simulink model "RWcontrol"  (R2022a)
settings: Solver=VariableStepAuto  StartTime=0.0  StopTime=10.0  RelTol=1e-3
undefined symbols (not defined in the file): a, b, c, D, J, Kt, Ra, Tc
settings Model: Creator=sokse  LastModifiedBy=sokse

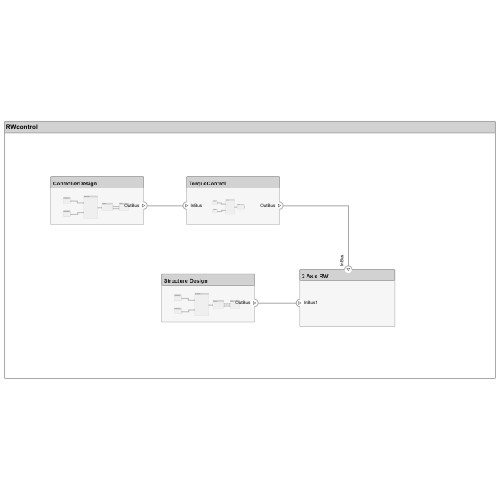
[thumbnail: Simulink's stored preview of the top-level diagram]
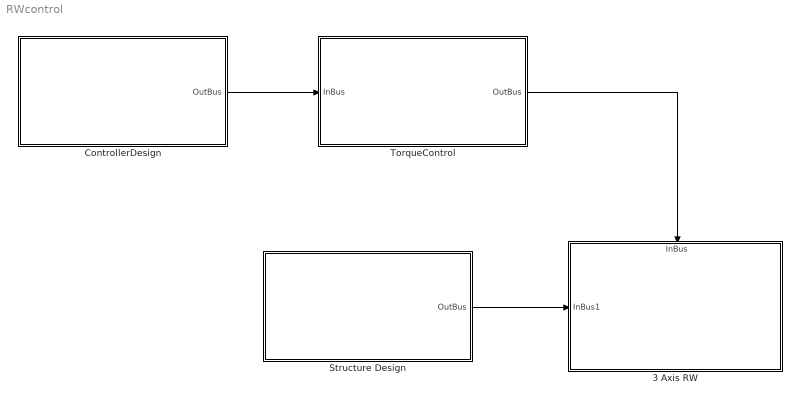
== system RWcontrol ==
  "3 Axis RW " : Subsystem
      settings: PortSchema="{\"entries\":[{\"content\":{\"headerSize\":26,\"margin\":15,\"minimumSpacing\":25,\"sides\":[{\"content\":{\"connectorIds\":[\"In1\"]},\"type\":\"ConnectorPlacement.EquallySpacedRectSide\",\"uuid\":\"5a3ed42f-ef60-4d5f-9f38-8a8f512792d6\"},{\"content\":{\"connectorIds\":[],\"side\":\"RIGHT\"},\"type\":\"ConnectorPlacement.EquallySpacedRectSide\",\"uuid\":\"59ceac5d-16f1-41c0-9a71-456f9fb7ce18\"},{\"content\":{\"connectorIds\":[\"In2\"],\"side\":\"TOP\"},\"type\":\"ConnectorPlacement.EquallySpacedRectSide\",\"uuid\":\"4a3f00af-2f72-40aa-9bae-562563b835ca\"}]},\"type\":\"ConnectorPlacement.EquallySpacedConnector\",\"uuid\":\"b5549df5-2814-423d-9e67-fe282ba68aba\"}],\"packageUris\":[\"http://schema.mathworks.com/mf0/Connector/R2020b\"],\"version\":\"1.0\"}"
  ControllerDesign : Subsystem
      settings: PortSchema="{\"entries\":[{\"content\":{\"headerSize\":26,\"margin\":15,\"minimumSpacing\":25,\"sides\":[{\"content\":{\"connectorIds\":[]},\"type\":\"ConnectorPlacement.EquallySpacedRectSide\",\"uuid\":\"5a3ed42f-ef60-4d5f-9f38-8a8f512792d6\"},{\"content\":{\"connectorIds\":[\"Out1\"],\"side\":\"RIGHT\"},\"type\":\"ConnectorPlacement.EquallySpacedRectSide\",\"uuid\":\"59ceac5d-16f1-41c0-9a71-456f9fb7ce18\"},{\"content\":{\"connectorIds\":[],\"side\":\"TOP\"},\"type\":\"ConnectorPlacement.EquallySpacedRectSide\",\"uuid\":\"4a3f00af-2f72-40aa-9bae-562563b835ca\"}]},\"type\":\"ConnectorPlacement.EquallySpacedConnector\",\"uuid\":\"b5549df5-2814-423d-9e67-fe282ba68aba\"}],\"packageUris\":[\"http://schema.mathworks.com/mf0/Connector/R2020b\"],\"version\":\"1.0\"}"
  Structure Design : Subsystem
      settings: PortSchema="{\"entries\":[{\"content\":{\"headerSize\":26,\"margin\":15,\"minimumSpacing\":25,\"sides\":[{\"content\":{\"connectorIds\":[]},\"type\":\"ConnectorPlacement.EquallySpacedRectSide\",\"uuid\":\"5a3ed42f-ef60-4d5f-9f38-8a8f512792d6\"},{\"content\":{\"connectorIds\":[\"Out1\"],\"side\":\"RIGHT\"},\"type\":\"ConnectorPlacement.EquallySpacedRectSide\",\"uuid\":\"59ceac5d-16f1-41c0-9a71-456f9fb7ce18\"},{\"content\":{\"connectorIds\":[],\"side\":\"TOP\"},\"type\":\"ConnectorPlacement.EquallySpacedRectSide\",\"uuid\":\"4a3f00af-2f72-40aa-9bae-562563b835ca\"}]},\"type\":\"ConnectorPlacement.EquallySpacedConnector\",\"uuid\":\"b5549df5-2814-423d-9e67-fe282ba68aba\"}],\"packageUris\":[\"http://schema.mathworks.com/mf0/Connector/R2020b\"],\"version\":\"1.0\"}"
  TorqueControl : Subsystem
      settings: PortSchema="{\"entries\":[{\"content\":{\"headerSize\":26,\"margin\":15,\"minimumSpacing\":25,\"sides\":[{\"content\":{\"connectorIds\":[\"In1\"]},\"type\":\"ConnectorPlacement.EquallySpacedRectSide\",\"uuid\":\"5a3ed42f-ef60-4d5f-9f38-8a8f512792d6\"},{\"content\":{\"connectorIds\":[\"Out1\"],\"side\":\"RIGHT\"},\"type\":\"ConnectorPlacement.EquallySpacedRectSide\",\"uuid\":\"59ceac5d-16f1-41c0-9a71-456f9fb7ce18\"},{\"content\":{\"connectorIds\":[],\"side\":\"TOP\"},\"type\":\"ConnectorPlacement.EquallySpacedRectSide\",\"uuid\":\"4a3f00af-2f72-40aa-9bae-562563b835ca\"}]},\"type\":\"ConnectorPlacement.EquallySpacedConnector\",\"uuid\":\"b5549df5-2814-423d-9e67-fe282ba68aba\"}],\"packageUris\":[\"http://schema.mathworks.com/mf0/Connector/R2020b\"],\"version\":\"1.0\"}"
  wires:
  ControllerDesign/1(OutBus) -> TorqueControl/1(InBus)
  TorqueControl/1(OutBus) -> "3 Axis RW "/2(InBus)
  Structure Design/1(OutBus) -> "3 Axis RW "/1(InBus1)

== system RWcontrol/3 Axis RW  ==
  Bus Element In2 : Inport  PortName=InBus1
  Bus Element In1 : Inport  Port=2  PortName=InBus

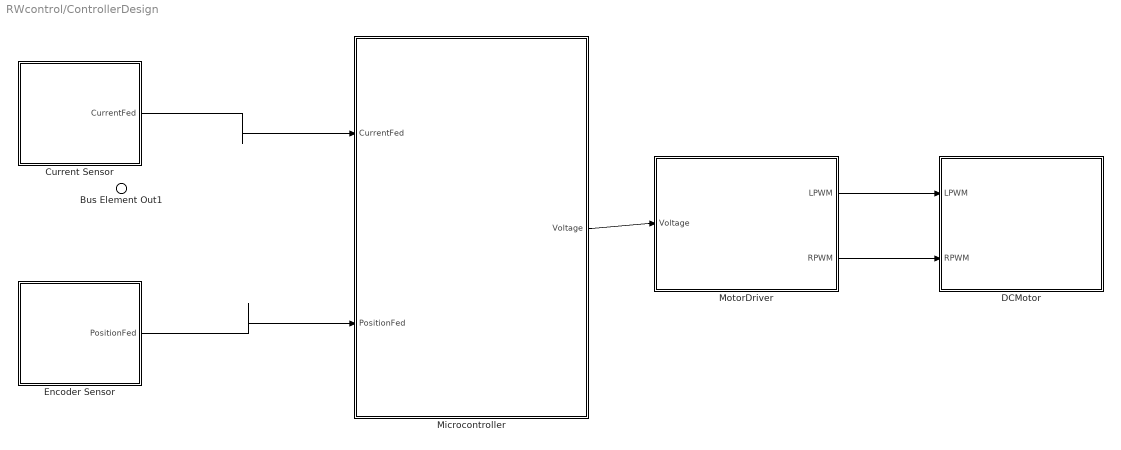
== system RWcontrol/ControllerDesign ==
  Current Sensor : Subsystem
      settings: PortSchema="{\"entries\":[{\"content\":{\"headerSize\":26,\"margin\":15,\"minimumSpacing\":25,\"sides\":[{\"content\":{\"connectorIds\":[]},\"type\":\"ConnectorPlacement.EquallySpacedRectSide\",\"uuid\":\"1e2ff6b6-1390-4131-a470-1fd24499352d\"},{\"content\":{\"connectorIds\":[\"Out1\"],\"side\":\"RIGHT\"},\"type\":\"ConnectorPlacement.EquallySpacedRectSide\",\"uuid\":\"b9c0b431-a60e-4bbb-a39b-9d90a7de03c4\"},{\"content\":{\"connectorIds\":[],\"side\":\"TOP\"},\"type\":\"ConnectorPlacement.EquallySpacedRectSide\",\"uuid\":\"16eb958a-beb2-45a6-99c7-d27e8684c515\"}]},\"type\":\"ConnectorPlacement.EquallySpacedConnector\",\"uuid\":\"784bec2e-ea8c-4097-8fb6-ddacd58b11f1\"}],\"packageUris\":[\"http://schema.mathworks.com/mf0/Connector/R2020b\"],\"version\":\"1.0\"}"
  "DCMotor " : Subsystem
      settings: PortSchema="{\"entries\":[{\"content\":{\"headerSize\":26,\"margin\":15,\"minimumSpacing\":25,\"sides\":[{\"content\":{\"connectorIds\":[\"In2\",\"In1\"]},\"type\":\"ConnectorPlacement.EquallySpacedRectSide\",\"uuid\":\"3b93c402-cac7-4c9a-af4f-66ab0cac09e6\"},{\"content\":{\"connectorIds\":[],\"side\":\"RIGHT\"},\"type\":\"ConnectorPlacement.EquallySpacedRectSide\",\"uuid\":\"1c6ece9f-2b60-418c-8344-c12dccd361a4\"},{\"content\":{\"connectorIds\":[],\"side\":\"TOP\"},\"type\":\"ConnectorPlacement.EquallySpacedRectSide\",\"uuid\":\"b9a36c11-6150-4268-84cd-3d41a85e6a91\"},{\"content\":{\"connectorIds\":[],\"side\":\"BOTTOM\"},\"type\":\"ConnectorPlacement.EquallySpacedRectSide\",\"uuid\":\"e2681d5f-5760-4ff1-ab06-0e137d65a698\"}]},\"type\":\"ConnectorPlacement.EquallySpacedConnector\",\"uuid\":\"82b2256f-f535-4640-b6be-fef3a7c38360\"}],\"packageUris\":[\"http://schema.mathworks.com/mf0/Connector/R2020b\"],\"version\":\"1.0\"}"
  Encoder Sensor : Subsystem
      settings: PortSchema="{\"entries\":[{\"content\":{\"headerSize\":26,\"margin\":15,\"minimumSpacing\":25,\"sides\":[{\"content\":{\"connectorIds\":[]},\"type\":\"ConnectorPlacement.EquallySpacedRectSide\",\"uuid\":\"1e2ff6b6-1390-4131-a470-1fd24499352d\"},{\"content\":{\"connectorIds\":[\"Out1\"],\"side\":\"RIGHT\"},\"type\":\"ConnectorPlacement.EquallySpacedRectSide\",\"uuid\":\"b9c0b431-a60e-4bbb-a39b-9d90a7de03c4\"},{\"content\":{\"connectorIds\":[],\"side\":\"TOP\"},\"type\":\"ConnectorPlacement.EquallySpacedRectSide\",\"uuid\":\"16eb958a-beb2-45a6-99c7-d27e8684c515\"}]},\"type\":\"ConnectorPlacement.EquallySpacedConnector\",\"uuid\":\"784bec2e-ea8c-4097-8fb6-ddacd58b11f1\"}],\"packageUris\":[\"http://schema.mathworks.com/mf0/Connector/R2020b\"],\"version\":\"1.0\"}"
  Microcontroller : Subsystem
      settings: PortSchema="{\"entries\":[{\"content\":{\"headerSize\":26,\"margin\":15,\"minimumSpacing\":25,\"sides\":[{\"content\":{\"connectorIds\":[\"In1\",\"In2\"]},\"type\":\"ConnectorPlacement.EquallySpacedRectSide\",\"uuid\":\"3b93c402-cac7-4c9a-af4f-66ab0cac09e6\"},{\"content\":{\"connectorIds\":[\"Out1\"],\"side\":\"RIGHT\"},\"type\":\"ConnectorPlacement.EquallySpacedRectSide\",\"uuid\":\"1c6ece9f-2b60-418c-8344-c12dccd361a4\"},{\"content\":{\"connectorIds\":[],\"side\":\"TOP\"},\"type\":\"ConnectorPlacement.EquallySpacedRectSide\",\"uuid\":\"b9a36c11-6150-4268-84cd-3d41a85e6a91\"}]},\"type\":\"ConnectorPlacement.EquallySpacedConnector\",\"uuid\":\"82b2256f-f535-4640-b6be-fef3a7c38360\"}],\"packageUris\":[\"http://schema.mathworks.com/mf0/Connector/R2020b\"],\"version\":\"1.0\"}"
  MotorDriver : Subsystem
      settings: PortSchema="{\"entries\":[{\"content\":{\"headerSize\":26,\"margin\":15,\"minimumSpacing\":25,\"sides\":[{\"content\":{\"connectorIds\":[\"In1\"]},\"type\":\"ConnectorPlacement.EquallySpacedRectSide\",\"uuid\":\"3b93c402-cac7-4c9a-af4f-66ab0cac09e6\"},{\"content\":{\"connectorIds\":[\"Out1\",\"Out2\"],\"side\":\"RIGHT\"},\"type\":\"ConnectorPlacement.EquallySpacedRectSide\",\"uuid\":\"1c6ece9f-2b60-418c-8344-c12dccd361a4\"},{\"content\":{\"connectorIds\":[],\"side\":\"TOP\"},\"type\":\"ConnectorPlacement.EquallySpacedRectSide\",\"uuid\":\"b9a36c11-6150-4268-84cd-3d41a85e6a91\"}]},\"type\":\"ConnectorPlacement.EquallySpacedConnector\",\"uuid\":\"82b2256f-f535-4640-b6be-fef3a7c38360\"}],\"packageUris\":[\"http://schema.mathworks.com/mf0/Connector/R2020b\"],\"version\":\"1.0\"}"
  Bus Element Out1 : Outport  PortName=OutBus
  wires:
  Current Sensor/1(CurrentFed) -> Microcontroller/1(CurrentFed)
  Encoder Sensor/1(PositionFed) -> Microcontroller/2(PositionFed)
  Microcontroller/1(Voltage) -> MotorDriver/1(Voltage)
  MotorDriver/1(LPWM) -> "DCMotor "/2(LPWM)
  MotorDriver/2(RPWM) -> "DCMotor "/1(RPWM)

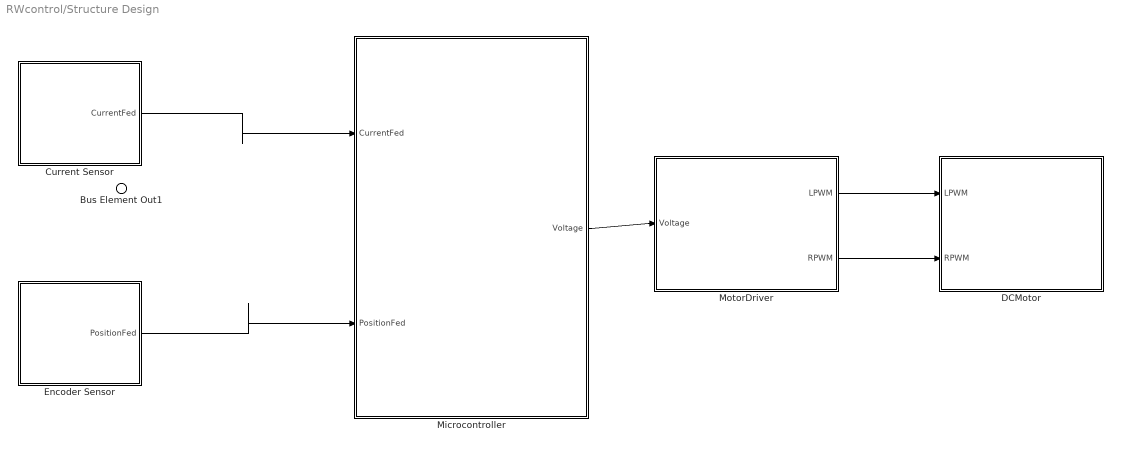
== system RWcontrol/Structure Design ==
  Current Sensor : Subsystem
      settings: PortSchema="{\"entries\":[{\"content\":{\"headerSize\":26,\"margin\":15,\"minimumSpacing\":25,\"sides\":[{\"content\":{\"connectorIds\":[]},\"type\":\"ConnectorPlacement.EquallySpacedRectSide\",\"uuid\":\"1e2ff6b6-1390-4131-a470-1fd24499352d\"},{\"content\":{\"connectorIds\":[\"Out1\"],\"side\":\"RIGHT\"},\"type\":\"ConnectorPlacement.EquallySpacedRectSide\",\"uuid\":\"b9c0b431-a60e-4bbb-a39b-9d90a7de03c4\"},{\"content\":{\"connectorIds\":[],\"side\":\"TOP\"},\"type\":\"ConnectorPlacement.EquallySpacedRectSide\",\"uuid\":\"16eb958a-beb2-45a6-99c7-d27e8684c515\"}]},\"type\":\"ConnectorPlacement.EquallySpacedConnector\",\"uuid\":\"784bec2e-ea8c-4097-8fb6-ddacd58b11f1\"}],\"packageUris\":[\"http://schema.mathworks.com/mf0/Connector/R2020b\"],\"version\":\"1.0\"}"
  "DCMotor " : Subsystem
      settings: PortSchema="{\"entries\":[{\"content\":{\"headerSize\":26,\"margin\":15,\"minimumSpacing\":25,\"sides\":[{\"content\":{\"connectorIds\":[\"In2\",\"In1\"]},\"type\":\"ConnectorPlacement.EquallySpacedRectSide\",\"uuid\":\"3b93c402-cac7-4c9a-af4f-66ab0cac09e6\"},{\"content\":{\"connectorIds\":[],\"side\":\"RIGHT\"},\"type\":\"ConnectorPlacement.EquallySpacedRectSide\",\"uuid\":\"1c6ece9f-2b60-418c-8344-c12dccd361a4\"},{\"content\":{\"connectorIds\":[],\"side\":\"TOP\"},\"type\":\"ConnectorPlacement.EquallySpacedRectSide\",\"uuid\":\"b9a36c11-6150-4268-84cd-3d41a85e6a91\"},{\"content\":{\"connectorIds\":[],\"side\":\"BOTTOM\"},\"type\":\"ConnectorPlacement.EquallySpacedRectSide\",\"uuid\":\"e2681d5f-5760-4ff1-ab06-0e137d65a698\"}]},\"type\":\"ConnectorPlacement.EquallySpacedConnector\",\"uuid\":\"82b2256f-f535-4640-b6be-fef3a7c38360\"}],\"packageUris\":[\"http://schema.mathworks.com/mf0/Connector/R2020b\"],\"version\":\"1.0\"}"
  Encoder Sensor : Subsystem
      settings: PortSchema="{\"entries\":[{\"content\":{\"headerSize\":26,\"margin\":15,\"minimumSpacing\":25,\"sides\":[{\"content\":{\"connectorIds\":[]},\"type\":\"ConnectorPlacement.EquallySpacedRectSide\",\"uuid\":\"1e2ff6b6-1390-4131-a470-1fd24499352d\"},{\"content\":{\"connectorIds\":[\"Out1\"],\"side\":\"RIGHT\"},\"type\":\"ConnectorPlacement.EquallySpacedRectSide\",\"uuid\":\"b9c0b431-a60e-4bbb-a39b-9d90a7de03c4\"},{\"content\":{\"connectorIds\":[],\"side\":\"TOP\"},\"type\":\"ConnectorPlacement.EquallySpacedRectSide\",\"uuid\":\"16eb958a-beb2-45a6-99c7-d27e8684c515\"}]},\"type\":\"ConnectorPlacement.EquallySpacedConnector\",\"uuid\":\"784bec2e-ea8c-4097-8fb6-ddacd58b11f1\"}],\"packageUris\":[\"http://schema.mathworks.com/mf0/Connector/R2020b\"],\"version\":\"1.0\"}"
  Microcontroller : Subsystem
      settings: PortSchema="{\"entries\":[{\"content\":{\"headerSize\":26,\"margin\":15,\"minimumSpacing\":25,\"sides\":[{\"content\":{\"connectorIds\":[\"In1\",\"In2\"]},\"type\":\"ConnectorPlacement.EquallySpacedRectSide\",\"uuid\":\"3b93c402-cac7-4c9a-af4f-66ab0cac09e6\"},{\"content\":{\"connectorIds\":[\"Out1\"],\"side\":\"RIGHT\"},\"type\":\"ConnectorPlacement.EquallySpacedRectSide\",\"uuid\":\"1c6ece9f-2b60-418c-8344-c12dccd361a4\"},{\"content\":{\"connectorIds\":[],\"side\":\"TOP\"},\"type\":\"ConnectorPlacement.EquallySpacedRectSide\",\"uuid\":\"b9a36c11-6150-4268-84cd-3d41a85e6a91\"}]},\"type\":\"ConnectorPlacement.EquallySpacedConnector\",\"uuid\":\"82b2256f-f535-4640-b6be-fef3a7c38360\"}],\"packageUris\":[\"http://schema.mathworks.com/mf0/Connector/R2020b\"],\"version\":\"1.0\"}"
  MotorDriver : Subsystem
      settings: PortSchema="{\"entries\":[{\"content\":{\"headerSize\":26,\"margin\":15,\"minimumSpacing\":25,\"sides\":[{\"content\":{\"connectorIds\":[\"In1\"]},\"type\":\"ConnectorPlacement.EquallySpacedRectSide\",\"uuid\":\"3b93c402-cac7-4c9a-af4f-66ab0cac09e6\"},{\"content\":{\"connectorIds\":[\"Out1\",\"Out2\"],\"side\":\"RIGHT\"},\"type\":\"ConnectorPlacement.EquallySpacedRectSide\",\"uuid\":\"1c6ece9f-2b60-418c-8344-c12dccd361a4\"},{\"content\":{\"connectorIds\":[],\"side\":\"TOP\"},\"type\":\"ConnectorPlacement.EquallySpacedRectSide\",\"uuid\":\"b9a36c11-6150-4268-84cd-3d41a85e6a91\"}]},\"type\":\"ConnectorPlacement.EquallySpacedConnector\",\"uuid\":\"82b2256f-f535-4640-b6be-fef3a7c38360\"}],\"packageUris\":[\"http://schema.mathworks.com/mf0/Connector/R2020b\"],\"version\":\"1.0\"}"
  Bus Element Out1 : Outport  PortName=OutBus
  wires:
  MotorDriver/2(RPWM) -> "DCMotor "/1(RPWM)
  MotorDriver/1(LPWM) -> "DCMotor "/2(LPWM)
  Microcontroller/1(Voltage) -> MotorDriver/1(Voltage)
  Encoder Sensor/1(PositionFed) -> Microcontroller/2(PositionFed)
  Current Sensor/1(CurrentFed) -> Microcontroller/1(CurrentFed)

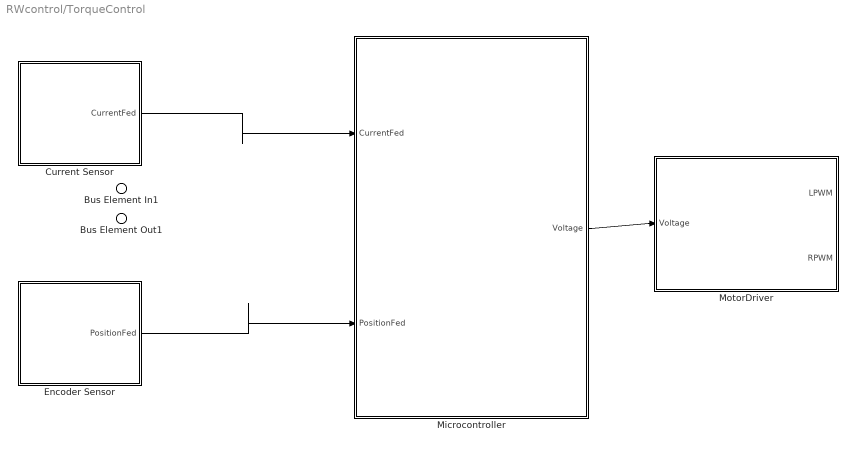
== system RWcontrol/TorqueControl ==
  Bus Element In1 : Inport  PortName=InBus
  Current Sensor : Subsystem
      settings: PortSchema="{\"entries\":[{\"content\":{\"headerSize\":26,\"margin\":15,\"minimumSpacing\":25,\"sides\":[{\"content\":{\"connectorIds\":[]},\"type\":\"ConnectorPlacement.EquallySpacedRectSide\",\"uuid\":\"1e2ff6b6-1390-4131-a470-1fd24499352d\"},{\"content\":{\"connectorIds\":[\"Out1\"],\"side\":\"RIGHT\"},\"type\":\"ConnectorPlacement.EquallySpacedRectSide\",\"uuid\":\"b9c0b431-a60e-4bbb-a39b-9d90a7de03c4\"},{\"content\":{\"connectorIds\":[],\"side\":\"TOP\"},\"type\":\"ConnectorPlacement.EquallySpacedRectSide\",\"uuid\":\"16eb958a-beb2-45a6-99c7-d27e8684c515\"}]},\"type\":\"ConnectorPlacement.EquallySpacedConnector\",\"uuid\":\"784bec2e-ea8c-4097-8fb6-ddacd58b11f1\"}],\"packageUris\":[\"http://schema.mathworks.com/mf0/Connector/R2020b\"],\"version\":\"1.0\"}"
  Encoder Sensor : Subsystem
      settings: PortSchema="{\"entries\":[{\"content\":{\"headerSize\":26,\"margin\":15,\"minimumSpacing\":25,\"sides\":[{\"content\":{\"connectorIds\":[]},\"type\":\"ConnectorPlacement.EquallySpacedRectSide\",\"uuid\":\"1e2ff6b6-1390-4131-a470-1fd24499352d\"},{\"content\":{\"connectorIds\":[\"Out1\"],\"side\":\"RIGHT\"},\"type\":\"ConnectorPlacement.EquallySpacedRectSide\",\"uuid\":\"b9c0b431-a60e-4bbb-a39b-9d90a7de03c4\"},{\"content\":{\"connectorIds\":[],\"side\":\"TOP\"},\"type\":\"ConnectorPlacement.EquallySpacedRectSide\",\"uuid\":\"16eb958a-beb2-45a6-99c7-d27e8684c515\"}]},\"type\":\"ConnectorPlacement.EquallySpacedConnector\",\"uuid\":\"784bec2e-ea8c-4097-8fb6-ddacd58b11f1\"}],\"packageUris\":[\"http://schema.mathworks.com/mf0/Connector/R2020b\"],\"version\":\"1.0\"}"
  Microcontroller : Subsystem
      settings: PortSchema="{\"entries\":[{\"content\":{\"headerSize\":26,\"margin\":15,\"minimumSpacing\":25,\"sides\":[{\"content\":{\"connectorIds\":[\"In1\",\"In2\"]},\"type\":\"ConnectorPlacement.EquallySpacedRectSide\",\"uuid\":\"3b93c402-cac7-4c9a-af4f-66ab0cac09e6\"},{\"content\":{\"connectorIds\":[\"Out1\"],\"side\":\"RIGHT\"},\"type\":\"ConnectorPlacement.EquallySpacedRectSide\",\"uuid\":\"1c6ece9f-2b60-418c-8344-c12dccd361a4\"},{\"content\":{\"connectorIds\":[],\"side\":\"TOP\"},\"type\":\"ConnectorPlacement.EquallySpacedRectSide\",\"uuid\":\"b9a36c11-6150-4268-84cd-3d41a85e6a91\"}]},\"type\":\"ConnectorPlacement.EquallySpacedConnector\",\"uuid\":\"82b2256f-f535-4640-b6be-fef3a7c38360\"}],\"packageUris\":[\"http://schema.mathworks.com/mf0/Connector/R2020b\"],\"version\":\"1.0\"}"
  MotorDriver : Subsystem
      settings: PortSchema="{\"entries\":[{\"content\":{\"headerSize\":26,\"margin\":15,\"minimumSpacing\":25,\"sides\":[{\"content\":{\"connectorIds\":[\"In1\"]},\"type\":\"ConnectorPlacement.EquallySpacedRectSide\",\"uuid\":\"3b93c402-cac7-4c9a-af4f-66ab0cac09e6\"},{\"content\":{\"connectorIds\":[\"Out1\",\"Out2\"],\"side\":\"RIGHT\"},\"type\":\"ConnectorPlacement.EquallySpacedRectSide\",\"uuid\":\"1c6ece9f-2b60-418c-8344-c12dccd361a4\"},{\"content\":{\"connectorIds\":[],\"side\":\"TOP\"},\"type\":\"ConnectorPlacement.EquallySpacedRectSide\",\"uuid\":\"b9a36c11-6150-4268-84cd-3d41a85e6a91\"}]},\"type\":\"ConnectorPlacement.EquallySpacedConnector\",\"uuid\":\"82b2256f-f535-4640-b6be-fef3a7c38360\"}],\"packageUris\":[\"http://schema.mathworks.com/mf0/Connector/R2020b\"],\"version\":\"1.0\"}"
  Bus Element Out1 : Outport  PortName=OutBus
  wires:
  Microcontroller/1(Voltage) -> MotorDriver/1(Voltage)
  Encoder Sensor/1(PositionFed) -> Microcontroller/2(PositionFed)
  Current Sensor/1(CurrentFed) -> Microcontroller/1(CurrentFed)

== system RWcontrol/ControllerDesign/Current Sensor ==
  Bus Element Out1 : Outport  PortName=CurrentFed

== system RWcontrol/ControllerDesign/DCMotor  ==
  Bus Element In1 : Inport  PortName=RPWM
  Bus Element In2 : Inport  Port=2  PortName=LPWM

== system RWcontrol/ControllerDesign/Encoder Sensor ==
  Bus Element Out1 : Outport  PortName=PositionFed

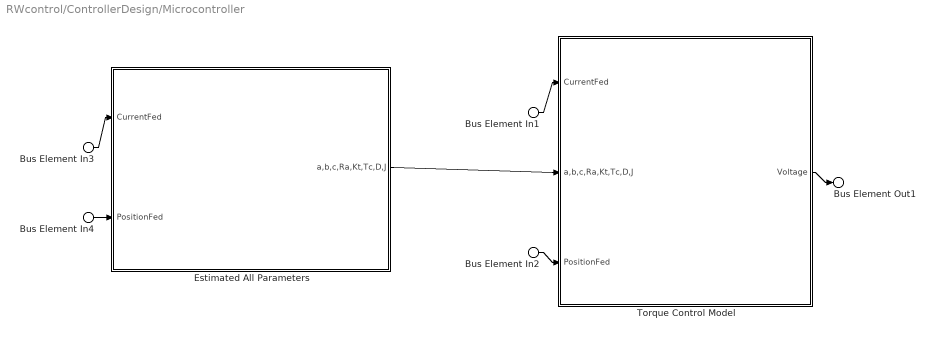
== system RWcontrol/ControllerDesign/Microcontroller ==
  Bus Element In1 : Inport  PortName=CurrentFed
  Bus Element In3 : Inport  PortName=CurrentFed
  Bus Element In2 : Inport  Port=2  PortName=PositionFed
  Bus Element In4 : Inport  Port=2  PortName=PositionFed
  Estimated All Parameters : Subsystem
      settings: PortSchema="{\"entries\":[{\"content\":{\"headerSize\":26,\"margin\":15,\"minimumSpacing\":25,\"sides\":[{\"content\":{\"connectorIds\":[\"In1\",\"In2\"]},\"type\":\"ConnectorPlacement.EquallySpacedRectSide\",\"uuid\":\"5a3ed42f-ef60-4d5f-9f38-8a8f512792d6\"},{\"content\":{\"connectorIds\":[\"Out1\"],\"side\":\"RIGHT\"},\"type\":\"ConnectorPlacement.EquallySpacedRectSide\",\"uuid\":\"59ceac5d-16f1-41c0-9a71-456f9fb7ce18\"},{\"content\":{\"connectorIds\":[],\"side\":\"TOP\"},\"type\":\"ConnectorPlacement.EquallySpacedRectSide\",\"uuid\":\"4a3f00af-2f72-40aa-9bae-562563b835ca\"}]},\"type\":\"ConnectorPlacement.EquallySpacedConnector\",\"uuid\":\"b5549df5-2814-423d-9e67-fe282ba68aba\"}],\"packageUris\":[\"http://schema.mathworks.com/mf0/Connector/R2020b\"],\"version\":\"1.0\"}"
  "Torque Control Model " : Subsystem
      settings: PortSchema="{\"entries\":[{\"content\":{\"headerSize\":26,\"margin\":15,\"minimumSpacing\":25,\"sides\":[{\"content\":{\"connectorIds\":[\"In1\",\"In2\",\"In3\"]},\"type\":\"ConnectorPlacement.EquallySpacedRectSide\",\"uuid\":\"1e2ff6b6-1390-4131-a470-1fd24499352d\"},{\"content\":{\"connectorIds\":[\"Out1\"],\"side\":\"RIGHT\"},\"type\":\"ConnectorPlacement.EquallySpacedRectSide\",\"uuid\":\"b9c0b431-a60e-4bbb-a39b-9d90a7de03c4\"},{\"content\":{\"connectorIds\":[],\"side\":\"TOP\"},\"type\":\"ConnectorPlacement.EquallySpacedRectSide\",\"uuid\":\"16eb958a-beb2-45a6-99c7-d27e8684c515\"}]},\"type\":\"ConnectorPlacement.EquallySpacedConnector\",\"uuid\":\"784bec2e-ea8c-4097-8fb6-ddacd58b11f1\"}],\"packageUris\":[\"http://schema.mathworks.com/mf0/Connector/R2020b\"],\"version\":\"1.0\"}"
  Bus Element Out1 : Outport  PortName=Voltage
  wires:
  Bus Element In4/1 -> Estimated All Parameters/2(PositionFed)
  Bus Element In3/1 -> Estimated All Parameters/1(CurrentFed)
  Estimated All Parameters/1(a,b,c,Ra,Kt,Tc,D,J) -> "Torque Control Model "/2(a,b,c,Ra,Kt,Tc,D,J)
  "Torque Control Model "/1(Voltage) -> Bus Element Out1/1
  Bus Element In1/1 -> "Torque Control Model "/1(CurrentFed)
  Bus Element In2/1 -> "Torque Control Model "/3(PositionFed)

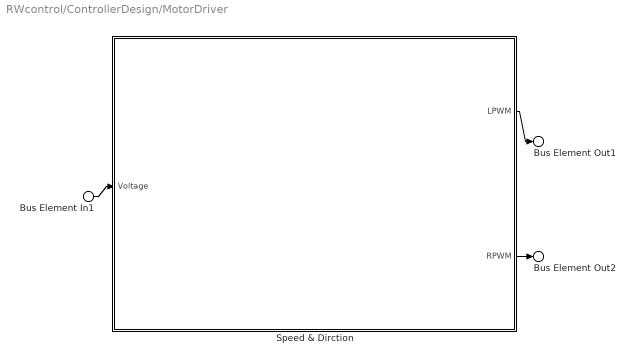
== system RWcontrol/ControllerDesign/MotorDriver ==
  Bus Element In1 : Inport  PortName=Voltage
  "Speed & Dirction " : Subsystem
      settings: PortSchema="{\"entries\":[{\"content\":{\"headerSize\":26,\"margin\":15,\"minimumSpacing\":25,\"sides\":[{\"content\":{\"connectorIds\":[\"In1\"]},\"type\":\"ConnectorPlacement.EquallySpacedRectSide\",\"uuid\":\"1e2ff6b6-1390-4131-a470-1fd24499352d\"},{\"content\":{\"connectorIds\":[\"Out1\",\"Out2\"],\"side\":\"RIGHT\"},\"type\":\"ConnectorPlacement.EquallySpacedRectSide\",\"uuid\":\"b9c0b431-a60e-4bbb-a39b-9d90a7de03c4\"},{\"content\":{\"connectorIds\":[],\"side\":\"TOP\"},\"type\":\"ConnectorPlacement.EquallySpacedRectSide\",\"uuid\":\"16eb958a-beb2-45a6-99c7-d27e8684c515\"}]},\"type\":\"ConnectorPlacement.EquallySpacedConnector\",\"uuid\":\"784bec2e-ea8c-4097-8fb6-ddacd58b11f1\"}],\"packageUris\":[\"http://schema.mathworks.com/mf0/Connector/R2020b\"],\"version\":\"1.0\"}"
  Bus Element Out1 : Outport  PortName=LPWM
  Bus Element Out2 : Outport  Port=2  PortName=RPWM
  wires:
  "Speed & Dirction "/2(RPWM) -> Bus Element Out2/1
  "Speed & Dirction "/1(LPWM) -> Bus Element Out1/1
  Bus Element In1/1 -> "Speed & Dirction "/1(Voltage)

== system RWcontrol/Structure Design/Current Sensor ==
  Bus Element Out1 : Outport  PortName=CurrentFed

== system RWcontrol/Structure Design/DCMotor  ==
  Bus Element In1 : Inport  PortName=RPWM
  Bus Element In2 : Inport  Port=2  PortName=LPWM

== system RWcontrol/Structure Design/Encoder Sensor ==
  Bus Element Out1 : Outport  PortName=PositionFed

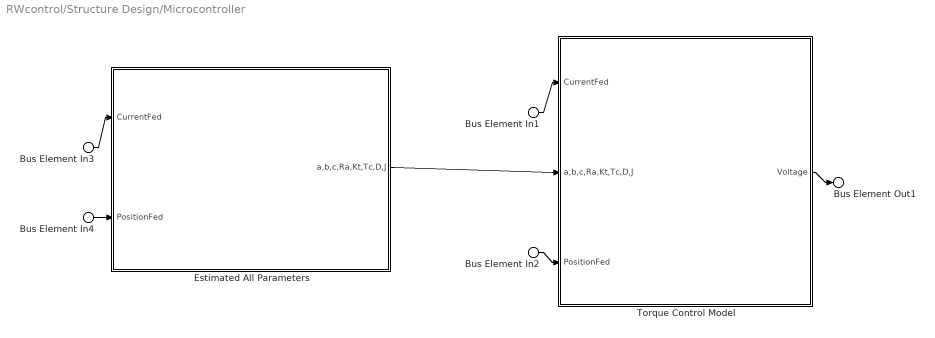
== system RWcontrol/Structure Design/Microcontroller ==
  Bus Element In1 : Inport  PortName=CurrentFed
  Bus Element In3 : Inport  PortName=CurrentFed
  Bus Element In2 : Inport  Port=2  PortName=PositionFed
  Bus Element In4 : Inport  Port=2  PortName=PositionFed
  Estimated All Parameters : Subsystem
      settings: PortSchema="{\"entries\":[{\"content\":{\"headerSize\":26,\"margin\":15,\"minimumSpacing\":25,\"sides\":[{\"content\":{\"connectorIds\":[\"In1\",\"In2\"]},\"type\":\"ConnectorPlacement.EquallySpacedRectSide\",\"uuid\":\"5a3ed42f-ef60-4d5f-9f38-8a8f512792d6\"},{\"content\":{\"connectorIds\":[\"Out1\"],\"side\":\"RIGHT\"},\"type\":\"ConnectorPlacement.EquallySpacedRectSide\",\"uuid\":\"59ceac5d-16f1-41c0-9a71-456f9fb7ce18\"},{\"content\":{\"connectorIds\":[],\"side\":\"TOP\"},\"type\":\"ConnectorPlacement.EquallySpacedRectSide\",\"uuid\":\"4a3f00af-2f72-40aa-9bae-562563b835ca\"}]},\"type\":\"ConnectorPlacement.EquallySpacedConnector\",\"uuid\":\"b5549df5-2814-423d-9e67-fe282ba68aba\"}],\"packageUris\":[\"http://schema.mathworks.com/mf0/Connector/R2020b\"],\"version\":\"1.0\"}"
  "Torque Control Model " : Subsystem
      settings: PortSchema="{\"entries\":[{\"content\":{\"headerSize\":26,\"margin\":15,\"minimumSpacing\":25,\"sides\":[{\"content\":{\"connectorIds\":[\"In1\",\"In2\",\"In3\"]},\"type\":\"ConnectorPlacement.EquallySpacedRectSide\",\"uuid\":\"1e2ff6b6-1390-4131-a470-1fd24499352d\"},{\"content\":{\"connectorIds\":[\"Out1\"],\"side\":\"RIGHT\"},\"type\":\"ConnectorPlacement.EquallySpacedRectSide\",\"uuid\":\"b9c0b431-a60e-4bbb-a39b-9d90a7de03c4\"},{\"content\":{\"connectorIds\":[],\"side\":\"TOP\"},\"type\":\"ConnectorPlacement.EquallySpacedRectSide\",\"uuid\":\"16eb958a-beb2-45a6-99c7-d27e8684c515\"}]},\"type\":\"ConnectorPlacement.EquallySpacedConnector\",\"uuid\":\"784bec2e-ea8c-4097-8fb6-ddacd58b11f1\"}],\"packageUris\":[\"http://schema.mathworks.com/mf0/Connector/R2020b\"],\"version\":\"1.0\"}"
  Bus Element Out1 : Outport  PortName=Voltage
  wires:
  Bus Element In2/1 -> "Torque Control Model "/3(PositionFed)
  Bus Element In1/1 -> "Torque Control Model "/1(CurrentFed)
  "Torque Control Model "/1(Voltage) -> Bus Element Out1/1
  Estimated All Parameters/1(a,b,c,Ra,Kt,Tc,D,J) -> "Torque Control Model "/2(a,b,c,Ra,Kt,Tc,D,J)
  Bus Element In3/1 -> Estimated All Parameters/1(CurrentFed)
  Bus Element In4/1 -> Estimated All Parameters/2(PositionFed)

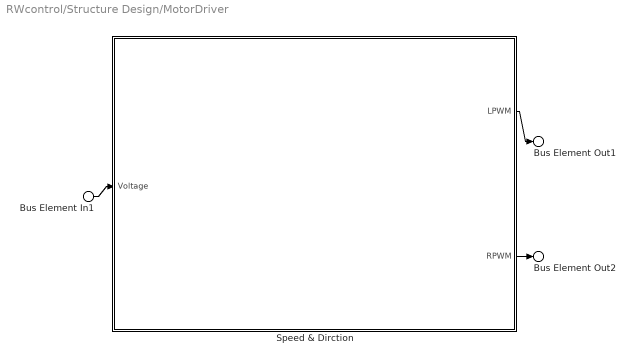
== system RWcontrol/Structure Design/MotorDriver ==
  Bus Element In1 : Inport  PortName=Voltage
  "Speed & Dirction " : Subsystem
      settings: PortSchema="{\"entries\":[{\"content\":{\"headerSize\":26,\"margin\":15,\"minimumSpacing\":25,\"sides\":[{\"content\":{\"connectorIds\":[\"In1\"]},\"type\":\"ConnectorPlacement.EquallySpacedRectSide\",\"uuid\":\"1e2ff6b6-1390-4131-a470-1fd24499352d\"},{\"content\":{\"connectorIds\":[\"Out1\",\"Out2\"],\"side\":\"RIGHT\"},\"type\":\"ConnectorPlacement.EquallySpacedRectSide\",\"uuid\":\"b9c0b431-a60e-4bbb-a39b-9d90a7de03c4\"},{\"content\":{\"connectorIds\":[],\"side\":\"TOP\"},\"type\":\"ConnectorPlacement.EquallySpacedRectSide\",\"uuid\":\"16eb958a-beb2-45a6-99c7-d27e8684c515\"}]},\"type\":\"ConnectorPlacement.EquallySpacedConnector\",\"uuid\":\"784bec2e-ea8c-4097-8fb6-ddacd58b11f1\"}],\"packageUris\":[\"http://schema.mathworks.com/mf0/Connector/R2020b\"],\"version\":\"1.0\"}"
  Bus Element Out1 : Outport  PortName=LPWM
  Bus Element Out2 : Outport  Port=2  PortName=RPWM
  wires:
  Bus Element In1/1 -> "Speed & Dirction "/1(Voltage)
  "Speed & Dirction "/1(LPWM) -> Bus Element Out1/1
  "Speed & Dirction "/2(RPWM) -> Bus Element Out2/1

== system RWcontrol/TorqueControl/Current Sensor ==
  Bus Element Out1 : Outport  PortName=CurrentFed

== system RWcontrol/TorqueControl/Encoder Sensor ==
  Bus Element Out1 : Outport  PortName=PositionFed

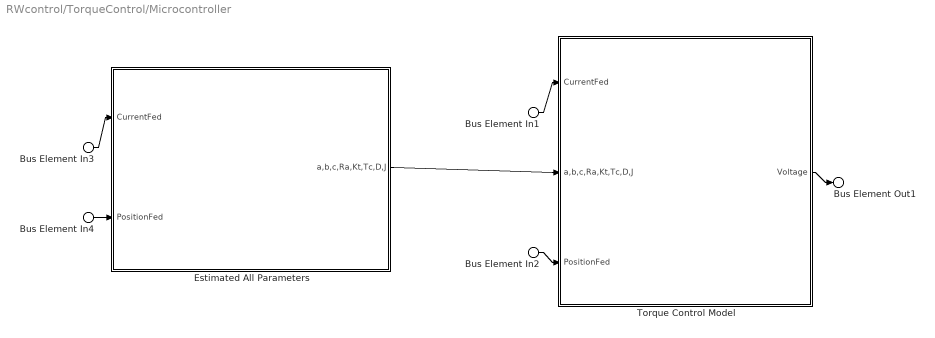
== system RWcontrol/TorqueControl/Microcontroller ==
  Bus Element In1 : Inport  PortName=CurrentFed
  Bus Element In3 : Inport  PortName=CurrentFed
  Bus Element In2 : Inport  Port=2  PortName=PositionFed
  Bus Element In4 : Inport  Port=2  PortName=PositionFed
  Estimated All Parameters : Subsystem
      settings: PortSchema="{\"entries\":[{\"content\":{\"headerSize\":26,\"margin\":15,\"minimumSpacing\":25,\"sides\":[{\"content\":{\"connectorIds\":[\"In1\",\"In2\"]},\"type\":\"ConnectorPlacement.EquallySpacedRectSide\",\"uuid\":\"5a3ed42f-ef60-4d5f-9f38-8a8f512792d6\"},{\"content\":{\"connectorIds\":[\"Out1\"],\"side\":\"RIGHT\"},\"type\":\"ConnectorPlacement.EquallySpacedRectSide\",\"uuid\":\"59ceac5d-16f1-41c0-9a71-456f9fb7ce18\"},{\"content\":{\"connectorIds\":[],\"side\":\"TOP\"},\"type\":\"ConnectorPlacement.EquallySpacedRectSide\",\"uuid\":\"4a3f00af-2f72-40aa-9bae-562563b835ca\"}]},\"type\":\"ConnectorPlacement.EquallySpacedConnector\",\"uuid\":\"b5549df5-2814-423d-9e67-fe282ba68aba\"}],\"packageUris\":[\"http://schema.mathworks.com/mf0/Connector/R2020b\"],\"version\":\"1.0\"}"
  "Torque Control Model " : Subsystem
      settings: PortSchema="{\"entries\":[{\"content\":{\"headerSize\":26,\"margin\":15,\"minimumSpacing\":25,\"sides\":[{\"content\":{\"connectorIds\":[\"In1\",\"In2\",\"In3\"]},\"type\":\"ConnectorPlacement.EquallySpacedRectSide\",\"uuid\":\"1e2ff6b6-1390-4131-a470-1fd24499352d\"},{\"content\":{\"connectorIds\":[\"Out1\"],\"side\":\"RIGHT\"},\"type\":\"ConnectorPlacement.EquallySpacedRectSide\",\"uuid\":\"b9c0b431-a60e-4bbb-a39b-9d90a7de03c4\"},{\"content\":{\"connectorIds\":[],\"side\":\"TOP\"},\"type\":\"ConnectorPlacement.EquallySpacedRectSide\",\"uuid\":\"16eb958a-beb2-45a6-99c7-d27e8684c515\"}]},\"type\":\"ConnectorPlacement.EquallySpacedConnector\",\"uuid\":\"784bec2e-ea8c-4097-8fb6-ddacd58b11f1\"}],\"packageUris\":[\"http://schema.mathworks.com/mf0/Connector/R2020b\"],\"version\":\"1.0\"}"
  Bus Element Out1 : Outport  PortName=Voltage
  wires:
  Bus Element In2/1 -> "Torque Control Model "/3(PositionFed)
  Bus Element In1/1 -> "Torque Control Model "/1(CurrentFed)
  "Torque Control Model "/1(Voltage) -> Bus Element Out1/1
  Estimated All Parameters/1(a,b,c,Ra,Kt,Tc,D,J) -> "Torque Control Model "/2(a,b,c,Ra,Kt,Tc,D,J)
  Bus Element In3/1 -> Estimated All Parameters/1(CurrentFed)
  Bus Element In4/1 -> Estimated All Parameters/2(PositionFed)

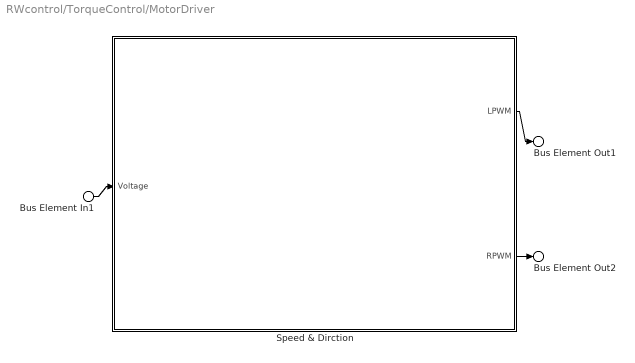
== system RWcontrol/TorqueControl/MotorDriver ==
  Bus Element In1 : Inport  PortName=Voltage
  "Speed & Dirction " : Subsystem
      settings: PortSchema="{\"entries\":[{\"content\":{\"headerSize\":26,\"margin\":15,\"minimumSpacing\":25,\"sides\":[{\"content\":{\"connectorIds\":[\"In1\"]},\"type\":\"ConnectorPlacement.EquallySpacedRectSide\",\"uuid\":\"1e2ff6b6-1390-4131-a470-1fd24499352d\"},{\"content\":{\"connectorIds\":[\"Out1\",\"Out2\"],\"side\":\"RIGHT\"},\"type\":\"ConnectorPlacement.EquallySpacedRectSide\",\"uuid\":\"b9c0b431-a60e-4bbb-a39b-9d90a7de03c4\"},{\"content\":{\"connectorIds\":[],\"side\":\"TOP\"},\"type\":\"ConnectorPlacement.EquallySpacedRectSide\",\"uuid\":\"16eb958a-beb2-45a6-99c7-d27e8684c515\"}]},\"type\":\"ConnectorPlacement.EquallySpacedConnector\",\"uuid\":\"784bec2e-ea8c-4097-8fb6-ddacd58b11f1\"}],\"packageUris\":[\"http://schema.mathworks.com/mf0/Connector/R2020b\"],\"version\":\"1.0\"}"
  Bus Element Out1 : Outport  PortName=LPWM
  Bus Element Out2 : Outport  Port=2  PortName=RPWM
  wires:
  Bus Element In1/1 -> "Speed & Dirction "/1(Voltage)
  "Speed & Dirction "/1(LPWM) -> Bus Element Out1/1
  "Speed & Dirction "/2(RPWM) -> Bus Element Out2/1

== system RWcontrol/ControllerDesign/Microcontroller/Estimated All Parameters ==
  Bus Element In1 : Inport  PortName=CurrentFed
  Bus Element In2 : Inport  Port=2  PortName=PositionFed
  Bus Element Out1 : Outport  PortName=a,b,c,Ra,Kt,Tc,D,J

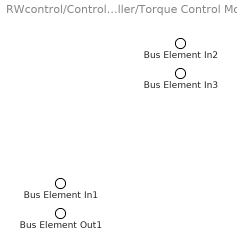
== system RWcontrol/ControllerDesign/Microcontroller/Torque Control Model  ==
  Bus Element In2 : Inport  PortName=CurrentFed
  Bus Element In3 : Inport  Port=2  PortName=a,b,c,Ra,Kt,Tc,D,J
  Bus Element In1 : Inport  Port=3  PortName=PositionFed
  Bus Element Out1 : Outport  PortName=Voltage

== system RWcontrol/ControllerDesign/MotorDriver/Speed & Dirction  ==
  Bus Element In1 : Inport  PortName=Voltage
  Bus Element Out1 : Outport  PortName=LPWM
  Bus Element Out2 : Outport  Port=2  PortName=RPWM

== system RWcontrol/Structure Design/Microcontroller/Estimated All Parameters ==
  Bus Element In1 : Inport  PortName=CurrentFed
  Bus Element In2 : Inport  Port=2  PortName=PositionFed
  Bus Element Out1 : Outport  PortName=a,b,c,Ra,Kt,Tc,D,J

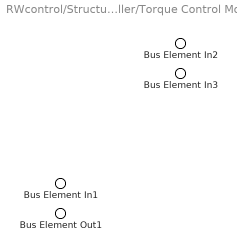
== system RWcontrol/Structure Design/Microcontroller/Torque Control Model  ==
  Bus Element In2 : Inport  PortName=CurrentFed
  Bus Element In3 : Inport  Port=2  PortName=a,b,c,Ra,Kt,Tc,D,J
  Bus Element In1 : Inport  Port=3  PortName=PositionFed
  Bus Element Out1 : Outport  PortName=Voltage

== system RWcontrol/Structure Design/MotorDriver/Speed & Dirction  ==
  Bus Element In1 : Inport  PortName=Voltage
  Bus Element Out1 : Outport  PortName=LPWM
  Bus Element Out2 : Outport  Port=2  PortName=RPWM

== system RWcontrol/TorqueControl/Microcontroller/Estimated All Parameters ==
  Bus Element In1 : Inport  PortName=CurrentFed
  Bus Element In2 : Inport  Port=2  PortName=PositionFed
  Bus Element Out1 : Outport  PortName=a,b,c,Ra,Kt,Tc,D,J

== system RWcontrol/TorqueControl/Microcontroller/Torque Control Model  ==
  Bus Element In2 : Inport  PortName=CurrentFed
  Bus Element In3 : Inport  Port=2  PortName=a,b,c,Ra,Kt,Tc,D,J
  Bus Element In1 : Inport  Port=3  PortName=PositionFed
  Bus Element Out1 : Outport  PortName=Voltage

== system RWcontrol/TorqueControl/MotorDriver/Speed & Dirction  ==
  Bus Element In1 : Inport  PortName=Voltage
  Bus Element Out1 : Outport  PortName=LPWM
  Bus Element Out2 : Outport  Port=2  PortName=RPWM
